simulink library "Lib_NM_JacobianCalc_TMATS"  (R2019b)
settings: Solver=ode45  StartTime=0.0  StopTime=10.0  RelTol=1e-3  EnableMultiTasking=on
Description:
  | Thomas Modules
settings Model: Creator=jwchapm2  LastModifiedBy=bhisma
settings DataIOCC: LimitDataPoints=on  SaveFormat=Array  ReturnWorkspaceOutputs=off
settings OptimizationCC: ExpressionDepthLimit=2147483647  LifeSpan=inf
settings DebuggingCC: UnderspecifiedInitializationDetection=Classic  MergeDetectMultiDrivingBlocksExec=none  SolverPrmCheckMsg=warning  StateNameClashWarn=warning  SFUnexpectedBacktrackingDiag=warning  SFNoUnconditionalDefaultTransitionDiag=warning  SFExecutionAtInitializationDiag=none  ArithmeticOperatorsInVariantConditions=warning
settings HardwareCC: ProdBitPerPointer=32  ProdBitPerSizeT=32  ProdBitPerPtrDiffT=32  ProdLargestAtomicFloat=None  ProdIntDivRoundTo=Undefined  ProdEndianess=Unspecified  ProdWordSize=32  ProdHWDeviceType=32-bit Generic
settings ModelReferenceCC: PropagateSignalLabelsOutOfModel=off
settings SFSimCC: SimUseLocalCustomCode=off  CustomCodeUndefinedFunction=UseInterfaceOnly
settings RTWCC: RTWUseLocalCustomCode=off
settings CodeAppCC: StateflowObjectComments=on
settings GRTTargetCC: TargetLangStandard=C89/C90 (ANSI)  GeneratePreprocessorConditionals=Disable all
settings ConfigComp: CovMetricSettings=dw  CovHtmlReporting=on  CovSaveCumulativeToWorkspaceVar=on  CovSaveSingleToWorkspaceVar=on  CovExternalEMLEnable=off

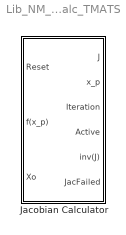
== system Lib_NM_JacobianCalc_TMATS ==
  Jacobian Calculator : Subsystem  TreatAsAtomicUnit=on  mask(T-MATS: Jacobian Calculator Library Block){N_Per_M=[0.01 0.01 0.01;-0.01 -0.01 -0.01]}
      mask prompts: N_Per_M "N_Per_M - Perturbations (nxm)"
      mask help:
      | The Jacobian Calculator block calculates the Jabobian of the system by perturbing the system around an initial point and calculating the gradient for each perturbation. This module will run once on start up and then again only if the reset is pressed.
      | Below: n (rows) is the number of times each independent will be perturbed and m (columns) is the number of inputs.
      mask Help: web(which('NumMthd_TMATS_JC.html'),'-helpbrowser')

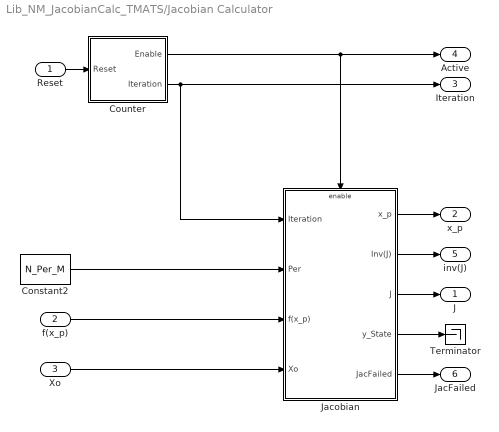
== system Lib_NM_JacobianCalc_TMATS/Jacobian Calculator ==
  Reset : Inport  PortDimensions=1
  f(x_p) : Inport  Port=2  PortDimensions=size(N_Per_M,2)
  Xo : Inport  Port=3  PortDimensions=size(N_Per_M,2)
  Constant2 : Constant  Value=N_Per_M
  Counter : Subsystem  mask{N_Ind_M=prod(size(N_Per_M))}
      mask prompts: N_Ind_M "number of independents, N_Ind_M"
  Jacobian : Subsystem
  Terminator : Terminator
  J : Outport  PortDimensions=[size(N_Per_M,2), size(N_Per_M,2)]
  x_p : Outport  Port=2  PortDimensions=size(N_Per_M,2)
  Iteration : Outport  Port=3  PortDimensions=1
  Active : Outport  Port=4  PortDimensions=1
  inv(J) : Outport  Port=5  PortDimensions=[size(N_Per_M,2), size(N_Per_M,2)]
  JacFailed : Outport  Port=6  PortDimensions=1
  wires:
  f(x_p)/1 -> Jacobian/3(f(x_p))
  Constant2/1 -> Jacobian/2(Per)
  Jacobian/1(x_p) -> x_p/1
  Reset/1 -> Counter/1(Reset)
  Counter/1(Enable) -> Active/1, Jacobian/Enable
  Xo/1 -> Jacobian/4(Xo)
  Counter/2(Iteration) -> Iteration/1, Jacobian/1(Iteration)
  Jacobian/2(Inv(J)) -> inv(J)/1
  Jacobian/3(J) -> J/1
  Jacobian/4(y_State) -> Terminator/1
  Jacobian/5(JacFailed) -> JacFailed/1

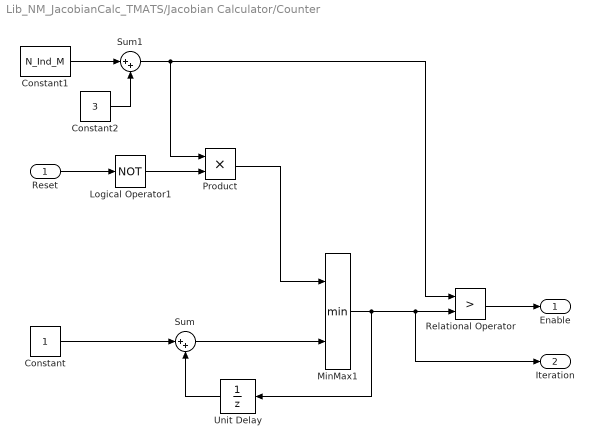
== system Lib_NM_JacobianCalc_TMATS/Jacobian Calculator/Counter ==
  Reset : Inport
  Constant : Constant
  Constant1 : Constant  Value=N_Ind_M
  Constant2 : Constant  Value=3
  Logical Operator1 : Logic  Operator=NOT  AllPortsSameDT=off  OutDataTypeStr=boolean
  MinMax1 : MinMax  Inputs=2
  Product : Product  RndMeth=Zero
  Relational Operator : RelationalOperator  Operator=>  OutDataTypeStr=boolean  RndMeth=Nearest
  Sum : Sum  Inputs=|++
  Sum1 : Sum  Inputs=|++
  Unit Delay : UnitDelay  SampleTime=-1  HasFrameUpgradeWarning=on
  Enable : Outport
  Iteration : Outport  Port=2
  wires:
  Constant/1 -> Sum/1
  Product/1 -> MinMax1/1
  Sum/1 -> MinMax1/2
  Unit Delay/1 -> Sum/2
  MinMax1/1 -> Unit Delay/1, Iteration/1, Relational Operator/2
  Relational Operator/1 -> Enable/1
  Logical Operator1/1 -> Product/2
  Reset/1 -> Logical Operator1/1
  Sum1/1 -> Relational Operator/1, Product/1
  Constant2/1 -> Sum1/2
  Constant1/1 -> Sum1/1

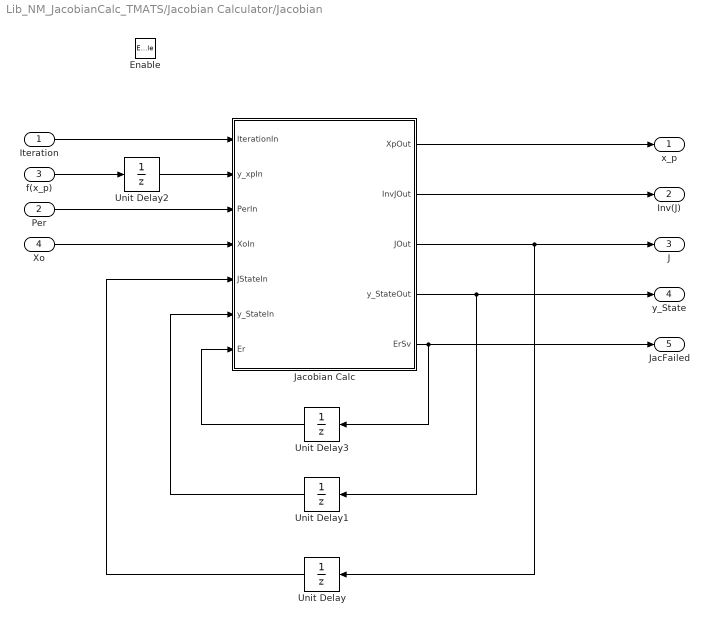
== system Lib_NM_JacobianCalc_TMATS/Jacobian Calculator/Jacobian ==
  Iteration : Inport
  Per : Inport  Port=2
  f(x_p) : Inport  Port=3
  Xo : Inport  Port=4
  Enable : EnablePort
  Jacobian Calc : MATLAB Function  TreatAsAtomicUnit=on
  Unit Delay : UnitDelay  InitialCondition=zeros(size(N_Per_M,2),size(N_Per_M,2))  SampleTime=-1  HasFrameUpgradeWarning=on
  Unit Delay1 : UnitDelay  InitialCondition=zeros(size(N_Per_M,2),prod(size(N_Per_M))+1)  SampleTime=-1  HasFrameUpgradeWarning=on
  Unit Delay2 : UnitDelay  InitialCondition=zeros(size(N_Per_M,2),1)  SampleTime=-1  HasFrameUpgradeWarning=on
  Unit Delay3 : UnitDelay  SampleTime=-1  HasFrameUpgradeWarning=on
  x_p : Outport
  Inv(J) : Outport  Port=2
  J : Outport  Port=3
  y_State : Outport  Port=4
  JacFailed : Outport  Port=5
  wires:
  Jacobian Calc/1(XpOut) -> x_p/1
  Xo/1 -> Jacobian Calc/4(XoIn)
  Per/1 -> Jacobian Calc/3(PerIn)
  Iteration/1 -> Jacobian Calc/1(IterationIn)
  Jacobian Calc/3(JOut) -> Unit Delay/1, J/1
  Jacobian Calc/2(InvJOut) -> Inv(J)/1
  Unit Delay/1 -> Jacobian Calc/5(JStateIn)
  Jacobian Calc/4(y_StateOut) -> Unit Delay1/1, y_State/1
  Unit Delay1/1 -> Jacobian Calc/6(y_StateIn)
  f(x_p)/1 -> Unit Delay2/1
  Unit Delay2/1 -> Jacobian Calc/2(y_xpIn)
  Jacobian Calc/5(ErSv) -> Unit Delay3/1, JacFailed/1
  Unit Delay3/1 -> Jacobian Calc/7(Er)

== matlab function Lib_NM_JacobianCalc_TMATS/Jacobian Calculator/Jacobian/Jacobian Calc ==
  data: IterationIn input; XpOut output; y_xpIn input; PerIn input; XoIn input; InvJOut output; JOut output; JStateIn input; y_StateIn input; y_StateOut output; Er input; ErSv output
function [XpOut, InvJOut, JOut, y_StateOut, ErSv] = fcn(IterationIn, y_xpIn, PerIn, XoIn, JStateIn, y_StateIn, Er)

% Set inital condiations
i = IterationIn;
XpOut = XoIn;
InvJOut = zeros(length(XoIn));
JOut = JStateIn;
y_StateOut = y_StateIn;
PerVec = reshape(PerIn',1,[]);
LenPV = length(PerVec);
LenXo = length(XoIn);
ErSv = Er;

% Begin taking data from f(x) at iteration a+1
a = 1;
% Begin determining Jacobian at iteration b+1
b = a+1;

% Set Xp Output
if i > a && i <= LenPV + a
    current_Xp = mod(i-a-1,LenXo)+1;
    XpOut(current_Xp) = XpOut(current_Xp) + PerVec(i - a);
end

% save state feedback
if LenXo == 1
    if i >= b;
        y_StateOut(i-a) = y_xpIn;
    end
else
    if i > a && i<= LenPV + a+1;
        y_StateOut(:,i - a) = y_xpIn;
    end
end

% Create Jacobian
if i == LenPV + b
    % Generate Jacobian matrices for each set, stacked.
    if LenXo == 1
        JMtx_extended = (y_StateOut(2:end)' - repmat(y_StateOut(1),1,LenPV))./PerVec;
    else
        JMtx_extended = (y_StateOut(:,2:end) - repmat(y_StateOut(:,1),1,LenPV))./repmat(PerVec,LenXo,1);
    end
    
    % Initialize sum matricies
    JMtrx_sum = zeros(LenXo);
    Nsum = zeros(LenXo);
    
    % determine how many perturbation sets there are, b/c MATLAB likes to
    % flip vectors when they enter MATLAB functions from Simulink for no reason.
    if min(size(PerIn)) == 1
     if LenXo == 1;
        PerNum = length(PerIn); 
     else 
        PerNum = 1;
     end
    else
        PerNum = size(PerIn,1);
    end
    
    for set = 1: PerNum
        % Break out Jacobian matrix for the current perturbation set
        JMtrx_cur = JMtx_extended(:, LenXo*(set-1)+1:LenXo*set);
        % Sum Jacobian matrices for each set
        JMtrx_sum = JMtrx_sum + JMtrx_cur(:,1:LenXo);
        % Sum number of acceptable values
        Nsum = Nsum + abs(sign(JMtrx_cur(:,1:LenXo)));
    end
    
    % Average Jacobian Matricies
    Javg = JMtrx_sum./max(Nsum,1);
    
    JOut = Javg;
    
    % Invert Jacobian
    if rank(JOut) == length(InvJOut)
        InvJOut = inv(JOut(:,:));
    elseif ErSv < 1
        disp('Jacobian can not be inverted.');
        ErSv = 1;
    end
end
